simulink model "last"  (R2024b)
settings: Solver=VariableStepAuto  StartTime=0.0  StopTime=10.0  RelTol=1e-3
undefined symbols (not defined in the file or in its folder): a_max, ia_limite, kamp, kdt, kff, ki, klim, kp, kt, kv, S_new2, T_regime1, Td1, Ts1, Vnom
libraries: cstblocks x2
settings Model: Creator=turco  LastModifiedBy=turco

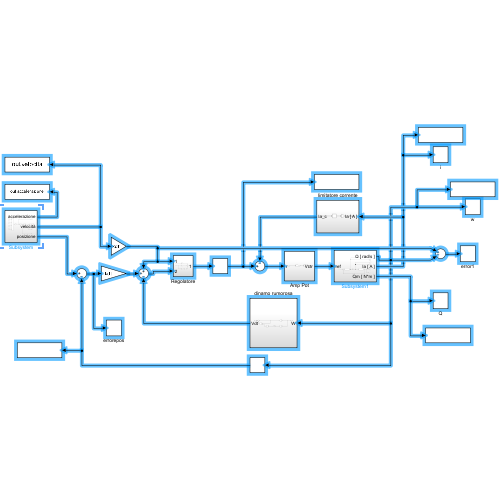
[thumbnail: Simulink's stored preview of the top-level diagram]
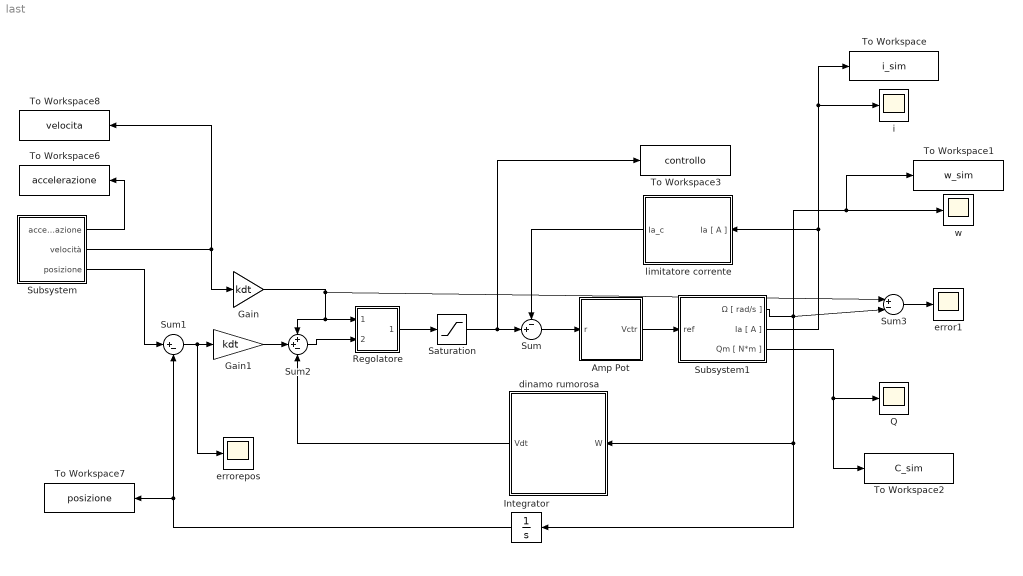
== system last ==
  Amp Pot : Subsystem
  Gain : Gain  Gain=kdt
  Gain1 : Gain  Gain=kdt
  Integrator : Integrator
  Q : Scope
  Regolatore : Subsystem
  Saturation : Saturate  UpperLimit=5  LowerLimit=-5
  Subsystem : Subsystem
  Subsystem1 : Subsystem
  Sum : Sum  Inputs=-+|
  Sum1 : Sum  Inputs=|+-
  Sum2 : Sum  Inputs=++-
  Sum3 : Sum  Inputs=|+-|
  To Workspace : ToWorkspace  VariableName=i_sim  SaveFormat=Timeseries  SampleTime=-1
  To Workspace1 : ToWorkspace  VariableName=w_sim  SaveFormat=Timeseries  SampleTime=-1
  To Workspace2 : ToWorkspace  VariableName=C_sim  SaveFormat=Timeseries  SampleTime=-1
  To Workspace3 : ToWorkspace  VariableName=controllo  SaveFormat=Timeseries  SampleTime=-1
  To Workspace6 : ToWorkspace  VariableName=accelerazione  SaveFormat=Timeseries  SampleTime=-1
  To Workspace7 : ToWorkspace  VariableName=posizione  SaveFormat=Timeseries  SampleTime=-1
  To Workspace8 : ToWorkspace  VariableName=velocita  SaveFormat=Timeseries  SampleTime=-1
  dinamo rumorosa : Subsystem
  error1 : Scope
  errorepos : Scope
  i : Scope
  limitatore corrente : Subsystem
  w : Scope
  wires:
  Subsystem1/3(Qm [ N*m ]) -> To Workspace2/1, Q/1
  Subsystem1/2(Ia [ A ]) -> To Workspace/1, i/1, limitatore corrente/1(Ia [ A ])
  Gain/1 -> Sum2/1, Regolatore/1(In1), Sum3/1
  Integrator/1 -> To Workspace7/1, Sum1/2
  Subsystem1/1(Ω [ rad/s ]) -> To Workspace1/1, w/1, Sum3/2, Integrator/1, dinamo rumorosa/1(W)
  Saturation/1 -> Sum/2, To Workspace3/1
  Subsystem/3(posizione) -> Sum1/1
  Subsystem/1(accelerazione) -> To Workspace6/1
  Sum/1 -> Amp Pot/1(r)
  Gain1/1 -> Sum2/2
  Sum2/1 -> Regolatore/2(In2)
  Regolatore/1(Out1) -> Saturation/1
  Subsystem/2(velocità) -> To Workspace8/1, Gain/1
  Amp Pot/1(Vctr) -> Subsystem1/1(ref)
  limitatore corrente/1(Ia_c) -> Sum/1
  Sum1/1 -> errorepos/1, Gain1/1
  dinamo rumorosa/1(Vdt) -> Sum2/3
  Sum3/1 -> error1/1

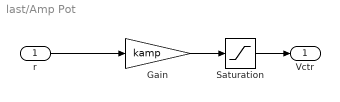
== system last/Amp Pot ==
  r : Inport
  Gain : Gain  Gain=kamp
  Saturation : Saturate  UpperLimit=+Vnom*1.2  LowerLimit=-Vnom*1.2
  Vctr : Outport
  wires:
  r/1 -> Gain/1
  Saturation/1 -> Vctr/1
  Gain/1 -> Saturation/1

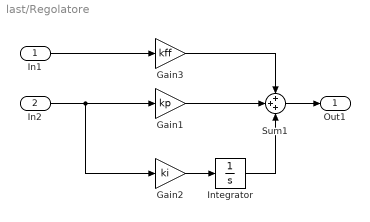
== system last/Regolatore ==
  In1 : Inport
  In2 : Inport  Port=2
  Gain1 : Gain  Gain=kp
  Gain2 : Gain  Gain=ki
  Gain3 : Gain  Gain=kff
  Integrator : Integrator  LimitOutput=on  UpperSaturationLimit=S_new2  LowerSaturationLimit=-S_new2
  Sum1 : Sum  Inputs=+++
  Out1 : Outport
  wires:
  In2/1 -> Gain2/1, Gain1/1
  Sum1/1 -> Out1/1
  In1/1 -> Gain3/1
  Integrator/1 -> Sum1/3
  Gain2/1 -> Integrator/1
  Gain1/1 -> Sum1/2
  Gain3/1 -> Sum1/1

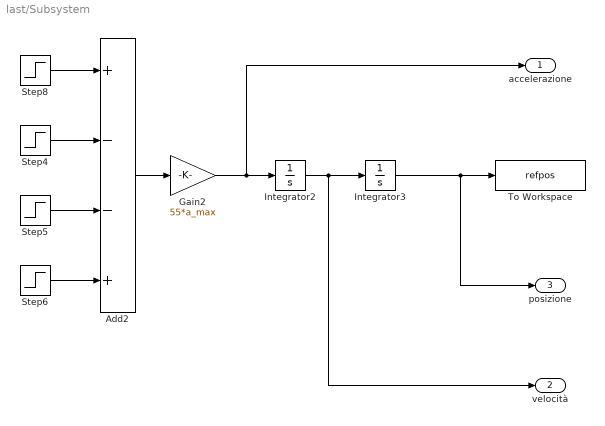
== system last/Subsystem ==
  Add2 : Sum  Inputs=+--+
  Gain2 : Gain  Gain=55*a_max
  Integrator2 : Integrator  UpperSaturationLimit=0.3707  LowerSaturationLimit=-0.3707
  Integrator3 : Integrator  UpperSaturationLimit=0.3707  LowerSaturationLimit=-0.3707
  Step4 : Step  Time=Ts1+0.2  SampleTime=0
  Step5 : Step  Time=Ts1+T_regime1+0.2  SampleTime=0
  Step6 : Step  Time=Ts1+T_regime1+Td1+0.2  SampleTime=0
  Step8 : Step  Time=0.2  SampleTime=0
  To Workspace : ToWorkspace  VariableName=refpos  SaveFormat=Timeseries  SampleTime=-1
  accelerazione : Outport
  velocità : Outport  Port=2
  posizione : Outport  Port=3
  wires:
  Step5/1 -> Add2/3
  Integrator3/1 -> posizione/1, To Workspace/1
  Step6/1 -> Add2/4
  Gain2/1 -> accelerazione/1, Integrator2/1
  Step4/1 -> Add2/2
  Add2/1 -> Gain2/1
  Step8/1 -> Add2/1
  Integrator2/1 -> velocità/1, Integrator3/1

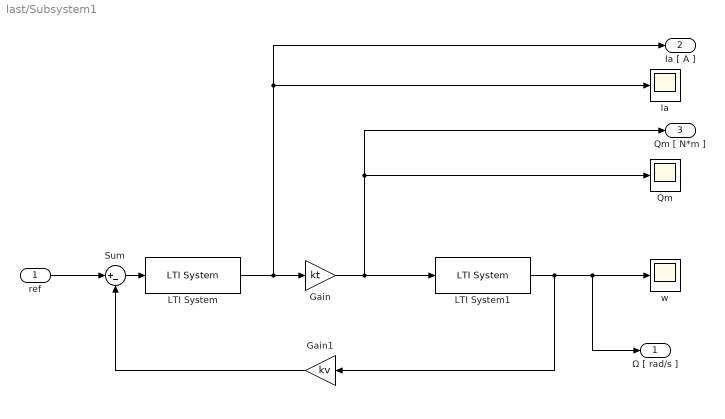
== system last/Subsystem1 ==
  ref : Inport
  Gain : Gain  Gain=kt
  Gain1 : Gain  Gain=kv
  Ia : Scope
  LTI System : cstblocks/LTI System  sys=Pel  IC=[]  PadeOrder=0
  LTI System1 : cstblocks/LTI System  sys=Pmec  IC=[]  PadeOrder=0
  "Qm " : Scope
  Sum : Sum  Inputs=|+-
  w : Scope
  Ω [ rad/s ] : Outport
  Ia [ A ] : Outport  Port=2
  Qm [ N*m ] : Outport  Port=3
  wires:
  LTI System1/1 -> Ω [ rad/s ]/1, w/1, Gain1/1
  Gain1/1 -> Sum/2
  Gain/1 -> Qm [ N*m ]/1, "Qm "/1, LTI System1/1
  Sum/1 -> LTI System/1
  LTI System/1 -> Ia [ A ]/1, Ia/1, Gain/1
  ref/1 -> Sum/1

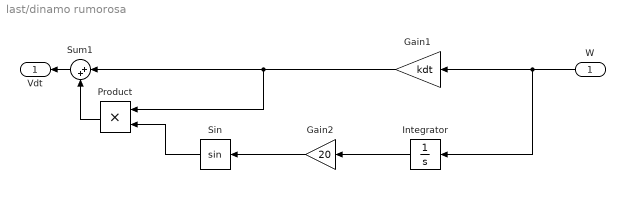
== system last/dinamo rumorosa ==
  W : Inport
  Gain1 : Gain  Gain=kdt
  Gain2 : Gain  Gain=20
  Integrator : Integrator
  Product : Product
  Sin : Trigonometry
  Sum1 : Sum  Inputs=|++
  Vdt : Outport
  wires:
  Integrator/1 -> Gain2/1
  Gain2/1 -> Sin/1
  W/1 -> Gain1/1, Integrator/1
  Product/1 -> Sum1/2
  Gain1/1 -> Product/1, Sum1/1
  Sin/1 -> Product/2
  Sum1/1 -> Vdt/1

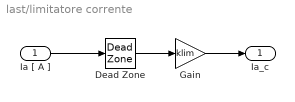
== system last/limitatore corrente ==
  Ia [ A ] : Inport
  Dead Zone : DeadZone  LowerValue=-ia_limite  UpperValue=+ia_limite
  Gain : Gain  Gain=klim
  Ia_c : Outport
  wires:
  Gain/1 -> Ia_c/1
  Ia [ A ]/1 -> Dead Zone/1
  Dead Zone/1 -> Gain/1
